simulink model "single_object"  (R2012b)
settings: Solver=ode3  StartTime=0.0  StopTime=simTime  FixedStep=stepSize  RelTol=1e-3
values from neighbouring files (symbols this model uses):
  delay = X(3)    [skrypt.m]
  den = [X(2) 1]    [skrypt.m]
  num = X(1)    [skrypt.m]
settings Model: Creator=Lao  LastModifiedBy=Lao

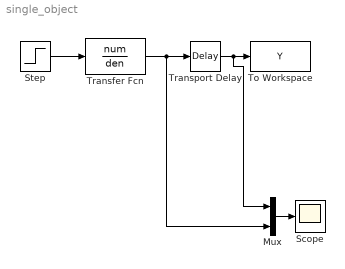
== system single_object ==
  Mux : Mux  Inputs=2
  Scope : Scope
  Step : Step  Time=0  SampleTime=0
  To Workspace : ToWorkspace  VariableName=Y  SampleTime=-1  SaveFormat=Structure With Time
  Transfer Fcn : TransferFcn  Numerator=num  Denominator=den
  Transport Delay : TransportDelay  DelayTime=delay  BufferSize=1000000
  wires:
  Step/1 -> Transfer Fcn/1
  Transfer Fcn/1 -> Mux/2, Transport Delay/1
  Transport Delay/1 -> Mux/1, To Workspace/1
  Mux/1 -> Scope/1
